simulink model "Mass_DigitalPID"  (R2016b)
settings: Solver=ode45  StartTime=0.0  StopTime=50  RelTol=1e-3  EnableMultiTasking=on
InitFcn:
  | param
undefined symbols (not defined in the file or in its folder): drawMassSys, mass_ctrl_state, P
settings Model: Creator=beard  LastModifiedBy=Jacob
settings DataIOCC: LimitDataPoints=on  SaveFormat=Array  SignalLoggingSaveFormat=ModelDataLogs
settings OptimizationCC: ExpressionDepthLimit=2147483647  InitFltsAndDblsToZero=on  LifeSpan=inf
settings DebuggingCC: UnderspecifiedInitializationDetection=Classic  MergeDetectMultiDrivingBlocksExec=none  SolverPrmCheckMsg=warning  FcnCallInpInsideContextMsg=warning  StateNameClashWarn=warning  SFUnexpectedBacktrackingDiag=warning  SFNoUnconditionalDefaultTransitionDiag=warning  SFExecutionAtInitializationDiag=none
settings HardwareCC: ProdBitPerPointer=32  ProdBitPerSizeT=32  ProdBitPerPtrDiffT=32  ProdLargestAtomicFloat=None  ProdIntDivRoundTo=Undefined  ProdEndianess=Unspecified  ProdWordSize=32  ProdHWDeviceType=32-bit Generic
settings ModelReferenceCC: PropagateSignalLabelsOutOfModel=off
settings GRTTargetCC: TargetLangStandard=C89/C90 (ANSI)  GeneratePreprocessorConditionals=Disable all  CombineOutputUpdateFcns=off  GRTInterface=on
settings ConfigComp: CovMetricSettings=dw  CovHtmlReporting=on  CovSaveCumulativeToWorkspaceVar=on  CovSaveSingleToWorkspaceVar=on  CovExternalEMLEnable=off

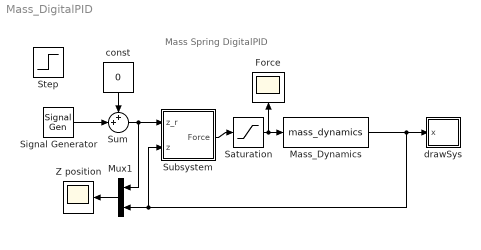
== system Mass_DigitalPID ==
  note: Mass Spring DigitalPID
  Force : Scope
  Mass_Dynamics : S-Function  FunctionName=mass_dynamics  Parameters=P  SFunctionDeploymentMode=off  EnableBusSupport=off
  Mux1 : Mux  Inputs=2
  Saturation : Saturate  UpperLimit=2  LowerLimit=-2
  Signal Generator : SignalGenerator  WaveForm=square  Amplitude=.5  Frequency=.03
  Step : Step  Time=0  After=.5  SampleTime=0
  Subsystem : Subsystem
  Sum : Sum  Inputs=++|
  Z position : Scope
  const : Constant  Value=0
  drawSys : Subsystem
  wires:
  Mass_Dynamics/1 -> Subsystem/2(z), Mux1/2, drawSys/1(x)
  Saturation/1 -> Force/1, Mass_Dynamics/1
  Mux1/1 -> Z position/1
  Subsystem/1(Force) -> Saturation/1
  Sum/1 -> Mux1/1, Subsystem/1(z_r)
  Signal Generator/1 -> Sum/2
  const/1 -> Sum/1

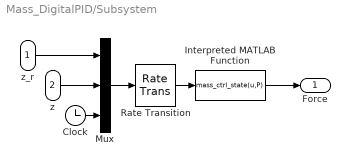
== system Mass_DigitalPID/Subsystem ==
  z_r : Inport
  z : Inport  Port=2
  Clock : Clock
  Interpreted MATLAB Function : MATLABFcn  MATLABFcn=mass_ctrl_state(u,P)
  Mux : Mux  Inputs=3
  Rate Transition : RateTransition  OutPortSampleTime=P.Ts
  Force : Outport
  wires:
  z_r/1 -> Mux/1
  z/1 -> Mux/2
  Mux/1 -> Rate Transition/1
  Rate Transition/1 -> Interpreted MATLAB Function/1
  Clock/1 -> Mux/3
  Interpreted MATLAB Function/1 -> Force/1

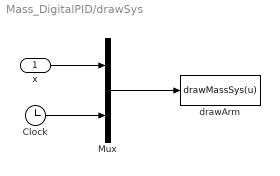
== system Mass_DigitalPID/drawSys ==
  x : Inport
  Clock : Clock
  Mux : Mux  Inputs=2
  drawArm : MATLABFcn  MATLABFcn=drawMassSys(u)  OutputDimensions=0  SampleTime=0.1
  wires:
  Mux/1 -> drawArm/1
  x/1 -> Mux/1
  Clock/1 -> Mux/2
